simulink subsystem "PvtSubSys_LATC"  (R2020b)
settings: Solver=VariableStepAuto  StartTime=0.0  StopTime=10.0  RelTol=1e-3
values from neighbouring files (symbols this model uses):
  P_Global_CharSpd_ms : value not decoded    [PubParsGlobal.sldd]
  P_Global_SteeringAngleRatio : value not decoded    [PubParsGlobal.sldd]
  P_Global_WheelBase_m : value not decoded    [PubParsGlobal.sldd]
  P_LCS_A0_Limit = 0.25    [LATC.sldd]    (also in LCS_v05.sldd)
  P_LCS_A1_Limit = 0.002    [LATC.sldd]    (also in LCS_v05.sldd)
  P_LCS_communicationTest = 1.0    [LATC.sldd]    (also in LCS_v05.sldd)
  P_LCS_Current_Offset_Test_SW = 0.0    [LATC.sldd]
  P_LCS_Current_Offset_Test_Value = 0.0    [LATC.sldd]
  P_LCS_Curvature_bp : value not decoded    [LATC.sldd]
  P_LCS_CycleTime = 0.4 0.4 0.4 0.4 0.4 0.4 0.4 0.4 0.4 0.6 0.6 0.6 0.6 0.6 0.6 0.6 0.4 0.4 0.4 0.4 0.4 0.4 0.4 0.4 0.4 0.6 0.6 0.6 0.6 0.6 0.6 0.6 0.4 0.4 0.4 0.4 0.4 0.4 0.4 0.4 0.4 0.6 0.6 0.6 0.6 0.6 0.6 0.6 0.4 0.4 0.4 0.4 0.4 0.4 0.4 0.4 0.4 0.6 0.6 0.6 0.6 0.6 0.6 0.6 0.4 0.4 0.4 0.4 0.4 0.4 0.4 0.4 0.4 0.6 0.6 0.6 0.6 0.6 0.6 0.6 0.4 0.4 0.4 0.4 0.4 0.4 0.4 0.4 0.4 0.6 0.6 0.6 0.6 0.6 0.6 0.6 0.4 0.4 0.4 0.4    [LATC.sldd]
  P_LCS_ESS_AngleSlope_Limit = 2.9    [LATC.sldd]    (also in LCS_v05.sldd)
  P_LCS_IN_Offset_Test_SW = 0.0    [LATC.sldd]    (also in LCS_v05.sldd)
  P_LCS_IN_Offset_Test_Value = 0.0    [LATC.sldd]    (also in LCS_v05.sldd)
  P_LCS_LATC_CurOffsetVehicleSpdLimitValue_degs = 7.0    [LATC.sldd]
  P_LCS_LATC_Du_Max = 20.0    [LATC.sldd]
  P_LCS_LATC_ELKAngleSlope_ratio : value not decoded    [LATC.sldd]
  P_LCS_LATC_ELKMaxLatAcc_ms2 : value not decoded    [LATC.sldd]
  P_LCS_LATC_ESSAngleSlope_ratio : value not decoded    [LATC.sldd]
  P_LCS_LATC_ESSMaxLatAcc_ms2 : value not decoded    [LATC.sldd]
  P_LCS_LATC_LCAngleSlope_ratio : value not decoded    [LATC.sldd]
  P_LCS_LATC_LCCancleMaxLatAcc_ms2 : value not decoded    [LATC.sldd]
  P_LCS_LATC_LCEcoAngleSlope_ratio : value not decoded    [LATC.sldd]
  P_LCS_LATC_LCEcoMaxLatAcc_ms2 : value not decoded    [LATC.sldd]
  P_LCS_LATC_LCKAngleSlope_ratio : value not decoded    [LATC.sldd]
  P_LCS_LATC_LCKIEAngleSlope_ratio : value not decoded    [LATC.sldd]
  P_LCS_LATC_LCKIEMaxLatAcc_ms2 : value not decoded    [LATC.sldd]
  P_LCS_LATC_LCKMaxLatAcc_ms2 : value not decoded    [LATC.sldd]
  P_LCS_LATC_LCNormalAngleSlope_ratio : value not decoded    [LATC.sldd]
  P_LCS_LATC_LCNormalMaxLatAcc_ms2 : value not decoded    [LATC.sldd]
  P_LCS_LATC_LCSportAngleSlope_ratio : value not decoded    [LATC.sldd]
  P_LCS_LATC_LCSportMaxLatAcc_ms2 : value not decoded    [LATC.sldd]
  P_LCS_LATC_LKAAngleSlope_ratio : value not decoded    [LATC.sldd]
  P_LCS_LATC_LKAMaxLatAcc_ms2 : value not decoded    [LATC.sldd]
  P_LCS_LATC_MatrixQ1_st = 0.8 0.8 1.2 1.4 1.4 1.4 2.0 2.2 2.2 2.2 2.2 2.2 2.2 2.2 2.2 2.2 0.8 0.8 1.2 1.4 1.4 1.4 2.0 2.2 2.2 2.2 2.2 2.2 2.2 2.2 2.2 2.2 0.8 0.8 1.2 1.4 1.4 1.4 2.0 2.2 2.2 2.2 2.2 2.2 2.2 2.2 2.2 2.2 0.8 0.8 1.2 1.4 1.4 1.4 2.0 2.2 2.2 2.2 2.2 2.2 2.2 2.2 2.2 2.2 0.8 0.8 1.2 1.4 1.4 1.4 2.0 2.2 2.2 2.2 2.2 2.2 2.2 2.2 2.2 2.2 0.8 0.8 1.2 1.4 1.4 1.4 2.0 2.2 2.2 2.2 2.2 2.2 2.2 2.2 2.2 2.2 0.8 0.8 1.2 1.4    [LATC.sldd]
  P_LCS_LATC_MatrixQ3_st = 20.0 20.0 20.0 20.0 20.0 15.0 15.0 15.0 15.0 15.0 15.0 15.0 15.0 13.0 13.0 13.0 20.0 20.0 20.0 20.0 20.0 15.0 15.0 15.0 15.0 15.0 15.0 15.0 15.0 13.0 13.0 13.0 20.0 20.0 20.0 20.0 20.0 15.0 15.0 15.0 15.0 15.0 15.0 15.0 15.0 13.0 13.0 13.0 20.0 20.0 20.0 20.0 20.0 15.0 15.0 15.0 15.0 15.0 15.0 15.0 15.0 13.0 13.0 13.0 20.0 20.0 20.0 20.0 20.0 15.0 15.0 15.0 15.0 15.0 15.0 15.0 15.0 13.0 13.0 13.0    [LATC.sldd]
  P_LCS_LATC_MatrixR_st = 10.0 10.0 10.0 10.0 10.0 10.0 10.0 15.0 15.0 15.0 15.0 15.0 15.0 15.0 15.0 15.0 10.0 10.0 10.0 10.0 10.0 10.0 10.0 15.0 15.0 15.0 15.0 15.0 15.0 15.0 15.0 15.0 10.0 10.0 10.0 10.0 10.0 10.0 10.0 15.0 15.0 15.0 15.0 15.0 15.0 15.0 15.0 15.0 10.0 10.0 10.0 10.0 10.0 10.0 10.0 15.0 15.0 15.0 15.0 15.0 15.0 15.0 15.0 15.0 10.0 10.0 10.0 10.0 10.0 10.0 10.0 15.0 15.0 15.0 15.0 15.0 15.0 15.0 15.0 15.0    [LATC.sldd]
  P_LCS_LATC_Max_LatAcc = 4.0    [LATC.sldd]
  P_LCS_LATC_Max_Phi = 15.0    [LATC.sldd]
  P_LCS_LATC_Max_y = 0.5    [LATC.sldd]
  P_LCS_LATC_MPC_SW = 0.0    [LATC.sldd]
  P_LCS_LATC_PreView_SW = 1.0    [LATC.sldd]
  P_LCS_LATC_SoftConstWeight = 1.0    [LATC.sldd]
  P_LCS_LATC_StateActivAngleSlopeLimit_ratio : value not decoded    [LATC.sldd]
  P_LCS_LATC_StateActiveFlg_TabX_st : value not decoded    [LATC.sldd]
  P_LCS_LATC_StateActiveHoldTime_TabY_st : value not decoded    [LATC.sldd]
  P_LCS_LATC_StateHoldTime_st = 250.0    [LATC.sldd]
  P_LCS_LATC_TarAngleFliterWindowSize = 5.0    [LATC.sldd]
  P_LCS_LATC_TarAngleLP_Time = 0.02    [LATC.sldd]
  P_LCS_LATC_U_Max = 90.0    [LATC.sldd]
  P_LCS_LCK_AngleSlope_Limit = 1.4    [LATC.sldd]
  P_LCS_LineVaildSW = 0.0    [LATC.sldd]
  P_LCS_Lookahead_Distance : value not decoded    [LATC.sldd]
  P_LCS_Lookahead_DistanceFac : value not decoded    [LATC.sldd]
  P_LCS_PLAN_CurvePreView_s = 0.3    [LATC.sldd]
  P_LCS_PLAN_CurvePreview_TabX_m : value not decoded    [LATC.sldd]
  P_LCS_PLAN_CurvePreViewFilterTime_s = 0.1    [LATC.sldd]
  P_LCS_PLAN_ELKAyDtLimit_Tab_ms3 = 1.0 1.0 1.0 1.0 1.0 1.0 1.0 1.0 1.0 1.0 1.0 1.0 1.0 1.0 1.0 1.0 1.0 1.0 1.0 1.0 1.0 1.0 1.0 1.0 1.0 1.0 1.0 1.0 1.0 1.0 1.0 1.0 1.0 1.0 1.0 1.0 1.0 1.0 1.0 1.0 1.0 1.0 1.0 1.0 1.0 1.0 1.0 1.0 1.0 1.0 1.0 1.0 1.0 1.0 1.0 1.0 1.0 1.0 1.0 1.0 1.0 1.0 1.0 1.0 1.0 1.0 1.0 1.0 1.0 1.0 1.0 1.0 1.0 1.0 1.0 1.0 1.0 1.0 1.0 1.0 1.0 1.0 1.0 1.0 1.0 1.0 1.0 1.0 1.0 1.0 1.0 1.0 1.0 1.0 1.0 1.0 1.0 1.0 1.0 1.0    [LATC.sldd]
  P_LCS_PLAN_ESSAyDtLimit_Tab_ms3 = 1.0 1.0 1.0 1.0 1.0 1.0 1.0 1.0 1.0 1.0 1.0 1.0 1.0 1.0 1.0 1.0 1.0 1.0 1.0 1.0 1.0 1.0 1.0 1.0 1.0 1.0 1.0 1.0 1.0 1.0 1.0 1.0 1.0 1.0 1.0 1.0 1.0 1.0 1.0 1.0 1.0 1.0 1.0 1.0 1.0 1.0 1.0 1.0 1.0 1.0 1.0 1.0 1.0 1.0 1.0 1.0 1.0 1.0 1.0 1.0 1.0 1.0 1.0 1.0 1.0 1.0 1.0 1.0 1.0 1.0 1.0 1.0 1.0 1.0 1.0 1.0 1.0 1.0 1.0 1.0 1.0 1.0 1.0 1.0 1.0 1.0 1.0 1.0 1.0 1.0 1.0 1.0 1.0 1.0 1.0 1.0 1.0 1.0 1.0 1.0    [LATC.sldd]
  P_LCS_PLAN_LCCancleAyDtLimit_Tab_ms3 = 1.0 1.0 1.0 1.0 1.0 1.0 1.0 1.0 1.0 1.0 1.0 1.0 1.0 1.0 1.0 1.0 1.0 1.0 1.0 1.0 1.0 1.0 1.0 1.0 1.0 1.0 1.0 1.0 1.0 1.0 1.0 1.0 1.0 1.0 1.0 1.0 1.0 1.0 1.0 1.0 1.0 1.0 1.0 1.0 1.0 1.0 1.0 1.0 1.0 1.0 1.0 1.0 1.0 1.0 1.0 1.0 1.0 1.0 1.0 1.0 1.0 1.0 1.0 1.0 1.0 1.0 1.0 1.0 1.0 1.0 1.0 1.0 1.0 1.0 1.0 1.0 1.0 1.0 1.0 1.0 1.0 1.0 1.0 1.0 1.0 1.0 1.0 1.0 1.0 1.0 1.0 1.0 1.0 1.0 1.0 1.0 1.0 1.0 1.0 1.0    [LATC.sldd]
  P_LCS_PLAN_LCEcoAyDtLimit_Tab_ms3 = 1.0 1.0 1.0 1.0 1.0 1.0 1.0 1.0 1.0 1.0 1.0 1.0 1.0 1.0 1.0 1.0 1.0 1.0 1.0 1.0 1.0 1.0 1.0 1.0 1.0 1.0 1.0 1.0 1.0 1.0 1.0 1.0 1.0 1.0 1.0 1.0 1.0 1.0 1.0 1.0 1.0 1.0 1.0 1.0 1.0 1.0 1.0 1.0 1.0 1.0 1.0 1.0 1.0 1.0 1.0 1.0 1.0 1.0 1.0 1.0 1.0 1.0 1.0 1.0 1.0 1.0 1.0 1.0 1.0 1.0 1.0 1.0 1.0 1.0 1.0 1.0 1.0 1.0 1.0 1.0 1.0 1.0 1.0 1.0 1.0 1.0 1.0 1.0 1.0 1.0 1.0 1.0 1.0 1.0 1.0 1.0 1.0 1.0 1.0 1.0    [LATC.sldd]
  P_LCS_PLAN_LCKAyDtLimit_Tab_ms3 = 1.5 1.5 1.5 1.5 1.5 1.5 1.5 1.5 1.5 1.5 1.5 1.5 1.5 1.5 1.5 1.5 1.5 1.5 1.5 1.5 1.5 1.5 1.5 1.5 1.5 1.5 1.5 1.5 1.5 1.5 1.5 1.5 1.5 1.5 1.5 1.5 1.5 1.5 1.5 1.5 1.5 1.5 1.5 1.5 1.5 1.5 1.5 1.5 1.5 1.5 1.5 1.5 1.5 1.5 1.5 1.5 1.5 1.5 1.5 1.5 1.5 1.5 1.5 1.5 1.5 1.5 1.5 1.5 1.5 1.5 1.5 1.5 1.5 1.5 1.5 1.5 1.5 1.5 1.5 1.5 1.5 1.5 1.5 1.5 1.5 1.5 1.5 1.5 1.5 1.5 1.5 1.5 1.5 1.5 1.5 1.5 1.5 1.5 1.5 1.5    [LATC.sldd]
  P_LCS_PLAN_LCKIEAyDtLimit_Tab_ms3 = 1.0 1.0 1.0 1.0 1.0 1.0 1.0 1.0 1.0 1.0 1.0 1.0 1.0 1.0 1.0 1.0 1.0 1.0 1.0 1.0 1.0 1.0 1.0 1.0 1.0 1.0 1.0 1.0 1.0 1.0 1.0 1.0 1.0 1.0 1.0 1.0 1.0 1.0 1.0 1.0 1.0 1.0 1.0 1.0 1.0 1.0 1.0 1.0 1.0 1.0 1.0 1.0 1.0 1.0 1.0 1.0 1.0 1.0 1.0 1.0 1.0 1.0 1.0 1.0 1.0 1.0 1.0 1.0 1.0 1.0 1.0 1.0 1.0 1.0 1.0 1.0 1.0 1.0 1.0 1.0 1.0 1.0 1.0 1.0 1.0 1.0 1.0 1.0 1.0 1.0 1.0 1.0 1.0 1.0 1.0 1.0 1.0 1.0 1.0 1.0    [LATC.sldd]
  P_LCS_PLAN_LCNormalAyDtLimit_Tab_ms3 = 1.0 1.0 1.0 1.0 1.0 1.0 1.0 1.0 1.0 1.0 1.0 1.0 1.0 1.0 1.0 1.0 1.0 1.0 1.0 1.0 1.0 1.0 1.0 1.0 1.0 1.0 1.0 1.0 1.0 1.0 1.0 1.0 1.0 1.0 1.0 1.0 1.0 1.0 1.0 1.0 1.0 1.0 1.0 1.0 1.0 1.0 1.0 1.0 1.0 1.0 1.0 1.0 1.0 1.0 1.0 1.0 1.0 1.0 1.0 1.0 1.0 1.0 1.0 1.0 1.0 1.0 1.0 1.0 1.0 1.0 1.0 1.0 1.0 1.0 1.0 1.0 1.0 1.0 1.0 1.0 1.0 1.0 1.0 1.0 1.0 1.0 1.0 1.0 1.0 1.0 1.0 1.0 1.0 1.0 1.0 1.0 1.0 1.0 1.0 1.0    [LATC.sldd]
  P_LCS_PLAN_LCSportAyDtLimit_Tab_ms3 = 1.0 1.0 1.0 1.0 1.0 1.0 1.0 1.0 1.0 1.0 1.0 1.0 1.0 1.0 1.0 1.0 1.0 1.0 1.0 1.0 1.0 1.0 1.0 1.0 1.0 1.0 1.0 1.0 1.0 1.0 1.0 1.0 1.0 1.0 1.0 1.0 1.0 1.0 1.0 1.0 1.0 1.0 1.0 1.0 1.0 1.0 1.0 1.0 1.0 1.0 1.0 1.0 1.0 1.0 1.0 1.0 1.0 1.0 1.0 1.0 1.0 1.0 1.0 1.0 1.0 1.0 1.0 1.0 1.0 1.0 1.0 1.0 1.0 1.0 1.0 1.0 1.0 1.0 1.0 1.0 1.0 1.0 1.0 1.0 1.0 1.0 1.0 1.0 1.0 1.0 1.0 1.0 1.0 1.0 1.0 1.0 1.0 1.0 1.0 1.0    [LATC.sldd]
  P_LCS_PLAN_LKAAyDtLimit_Tab_ms3 = 1.0 1.0 1.0 1.0 1.0 1.0 1.0 1.0 1.0 1.0 1.0 1.0 1.0 1.0 1.0 1.0 1.0 1.0 1.0 1.0 1.0 1.0 1.0 1.0 1.0 1.0 1.0 1.0 1.0 1.0 1.0 1.0 1.0 1.0 1.0 1.0 1.0 1.0 1.0 1.0 1.0 1.0 1.0 1.0 1.0 1.0 1.0 1.0 1.0 1.0 1.0 1.0 1.0 1.0 1.0 1.0 1.0 1.0 1.0 1.0 1.0 1.0 1.0 1.0 1.0 1.0 1.0 1.0 1.0 1.0 1.0 1.0 1.0 1.0 1.0 1.0 1.0 1.0 1.0 1.0 1.0 1.0 1.0 1.0 1.0 1.0 1.0 1.0 1.0 1.0 1.0 1.0 1.0 1.0 1.0 1.0 1.0 1.0 1.0 1.0    [LATC.sldd]
  P_LCS_PLAN_MinPlanDis_m : value not decoded    [LATC.sldd]
  P_LCS_PLAN_PreCurMinDisFac_ratio : value not decoded    [LATC.sldd]
  P_LCS_PLAN_PreDisCurve_TabX_m : value not decoded    [LATC.sldd]
  P_LCS_PLAN_StateActiv_AyDtLimit_ms3 : value not decoded    [LATC.sldd]
  P_LCS_PLAN_VehicleSpd_TabX_kph : value not decoded    [LATC.sldd]
  P_LCS_PLAN_VehicleSpd_TabY_Kph : value not decoded    [LATC.sldd]
  P_LCS_Trq_Switch = 0.0    [LATC.sldd]    (also in LCS_v05.sldd)
  P_LCS_VehicleSpd_TabX_Kph : value not decoded    [LATC.sldd]
undefined symbols (not defined in the file or in its folder): HWP_AngCmdReqVal, HWP_AngCmdReqValVld, HWP_FuncTrqCmdReqFlag, HWP_ReqCtrlEPS, HWP_ReqCtrlEPSVld, HWP_TrqOvlCmdReqValue, HWP_WorkReq, HWP_WorkReqVld
libraries: simulink x4, dspbuff3 x2
(part 6 of 8)

== matlab function PvtSubSys_LATC/LATC/LateralControl/LCS_Angle/Controller/TargetAngleCalc/TarSteerAngleCalc ==
  data: Final_steer_angle_cmd output; LatError_contribution output; LatErrorRate_contribution output; HeadingError_contribution output; HeadingErrorRate_contribution output; ControlValid input; SteerAngle input; CurrentSteerAngleOffset input; steer_angle_cmd output size=[1,1]; vy input; vx input; phi input; phi_dot input; TarTraj_x input size=[100 1]; TarTraj_y input size=[100 1]; Left_steer_ratio input; Right_steer_ratio input; Matrix_q1 input; Matrix_q2 input; Matrix_R input; Max_Phi input; Max_y input; U_Max input; Du_Max input; Max_LatAcc input; SoftConstWeight input
function [Final_steer_angle_cmd,LatError_contribution,LatErrorRate_contribution,...
    HeadingError_contribution,HeadingErrorRate_contribution,steer_angle_cmd]= ...
    MPC_ReferenceTrajectory_Algorithm(ControlValid,SteerAngle,CurrentSteerAngleOffset,vy,vx,phi,phi_dot,TarTraj_x,TarTraj_y,...
    Left_steer_ratio,Right_steer_ratio,Matrix_q1,Matrix_q2,Matrix_R,Max_Phi,Max_y,U_Max,Du_Max,Max_LatAcc,SoftConstWeight)

LatError_contribution = single(0);
LatErrorRate_contribution = single(0);
HeadingError_contribution = single(0);
HeadingErrorRate_contribution = single(0);
if ControlValid
    %% 1.车辆参数
    %1.1 车的大小及长度参数
    veh_params.vehicle_length = single(4.875);
    veh_params.vehicle_width  = single(2.2);
    veh_params.vehicle_height = single(1.69);
    %1.2 车辆控制参数
    veh_params.wheel_base = single(2.92);               %轴距, m
    veh_params.Vch = single(23.5);                      %特征车速
    veh_params.mu = single(0.85);                       %路面摩擦限制
    veh_params.max_acceleration = single(2);            %车辆最大加速度
    veh_params.max_deceleration = single(-2);           %车辆最大减速度
    veh_params.left_steer_ratio = Left_steer_ratio;     %车辆左侧转向传动比%
    veh_params.right_steer_ratio = Right_steer_ratio;   %车辆右侧转向传动比%
    veh_params.cf = single(55000);                      %车辆前轮侧偏刚度N/rad(两侧轮胎等效为一个*2)
    veh_params.cr = single(55000);                      %车辆后轮侧偏刚度N/rad
    veh_params.clf = single(5000);                      %车辆前轮纵向刚度(两侧轮胎等效为一个*2)
    veh_params.clr = single(5000);                      %车辆后轮纵向刚度
    
    veh_params.mass_fl = single(520);                   %车辆左前轮负重
    veh_params.mass_fr = single(520);                   %车辆右前轮负重
    veh_params.mass_rl = single(520);                   %车辆左后轮负重
    veh_params.mass_rr = single(520);                   %车辆右后轮负重
    veh_params.Sf = single(0.2);                        %车辆前轮滑移率
    veh_params.Sr = single(0.2);                        %车辆后轮滑移率
    %1.3 方向盘转角转换为车轮转角+度转弧度
    if (SteerAngle>=single(0))
        steer_transmission_ratio = veh_params.left_steer_ratio;
    else
        steer_transmission_ratio = veh_params.right_steer_ratio;
    end
    % FrontWheel_AngleK1_rad = steer_angleK1 / (single(57.3) * steer_transmission_ratio);%反算前轮转角并转换成弧度制 上一帧请求值
    FrontWheel_AngleK1_rad = SteerAngle/(single(57.3) * steer_transmission_ratio); %反算前轮转角并转换成弧度制
   %% 2.控制参数计算
    mass_front =  veh_params.mass_fl + veh_params.mass_fr;
    mass_rear  =  veh_params.mass_rl + veh_params.mass_rr;
    mass =  mass_front + mass_rear;
    lf = veh_params.wheel_base * (single(1.0) - mass_front / mass);% distance from front tires to cg, m 前轴到质心的距离
    lr = veh_params.wheel_base * (single(1.0) - mass_rear / mass);% distance from rear tires to cg, m  后轴到质心的距离
    iz = lf * lf * mass_front + lr * lr * mass_rear; % 转动惯量
    %---------------------------求车辆响应增益---------------------------%
    % % 车辆模型，状态为[beta,wr]
    % 求车辆响应增益
    Veh_Speed = (max(vx, single(0.2)));
    AAr = [(veh_params.cf+veh_params.cr),((veh_params.cf*lf-veh_params.cr*lr)/Veh_Speed)+mass*Veh_Speed;
           (veh_params.cf*lf-veh_params.cr*lr),(veh_params.cf*lf^2+veh_params.cr*lr^2)/Veh_Speed];
    BBr = [veh_params.cf;veh_params.cf*lf];
    a11 = AAr(1,1);
    a12 = AAr(1,2);
    a21 = AAr(2,1);
    a22 = AAr(2,2);
    b1 = BBr(1);
    b2 = BBr(2);
    %Ta = a11+a22;
    Da = a11*a22-a12*a21;
    
    Gr = (b2.*a11-b1.*a21)./Da;   % 稳态横摆角速度增益，理想化增益是偏大，因为轮胎侧偏刚度会变小
    % Gb = (b1.*a22-b2.*a12)./Da; % 稳态质心侧偏角增益，理想化增益是偏大，因为轮胎侧偏刚度会变小
    Gay = Gr*Veh_Speed;           % 稳态侧向加速度增益，理想化增益是偏大，因为轮胎侧偏刚度会变小
   %% 3.mpc算法
   % ----------------------车辆动力学模型--------------------------------%
   % 状态量=[y_dot,x_dot,phi,phi_dot,Y,X]，控制量为前轮偏角delta_f
   % dy_dot=-x_dot*phi_dot+2*(Ccf*(delta_f-(y_dot+a*phi_dot)/x_dot)+Ccr*(b*phi_dot-y_dot)/x_dot)/m;
   % dx_dot=y_dot*phi_dot+2*(Clf*Sf+Clr*Sr-Ccf*delta_f*(delta_f-(y_dot+phi_dot*a)/x_dot))/m;
   % dphi_dot=dphi_dot;
   % dphi_dot=(2*a*Ccf*(delta_f-(y_dot+a*phi_dot)/x_dot)-2*b*Ccr*(b*phi_dot-y_dot)/x_dot)/I;
   % Y_dot=x_dot*sin(phi)+y_dot*cos(phi);
   % X_dot=x_dot*cos(phi)-y_dot*sin(phi);
   % 通过Matlab求雅克比矩阵
   % 雅克比矩阵求解
   % f=[dy_dot;dx_dot;phi_dot;dphi_dot;Y_dot;X_dot];%动力学模型
   % kesi=[y_dot,x_dot,phi,phi_dot,Y,X];%系统状态量
   % v=delta_f;
   % R=jacobian(f,kesi);%矩阵A(t)-连续
   % R2=jacobian(f,v);%矩阵B(t)-连续
    A =  [-((2*veh_params.cf)/vx+(2*veh_params.cr)/vx)/mass   ((2*veh_params.cf*(vy+lf*phi_dot))/vx^2+(2*veh_params.cr*(vy-lr*phi_dot))/vx^2)/mass-phi_dot   0   -vx-((2*veh_params.cf*lf)/vx-(2*veh_params.cr*lr)/vx)/mass   0   0;
          phi_dot + (2*veh_params.cf*FrontWheel_AngleK1_rad)/(mass*vx)       -(2*veh_params.cf*FrontWheel_AngleK1_rad*(vy + lf*phi_dot))/(mass*vx^2)         0   vy + (2*veh_params.cf*lf*FrontWheel_AngleK1_rad)/(mass*vx)   0   0;
          0                                                    0                                                                                             0   1                                                            0   0;
    -((2*veh_params.cf*lf)/vx-(2*veh_params.cr*lr)/vx)/iz   ((2*veh_params.cf*lf*(vy+lf*phi_dot))/vx^2-(2*veh_params.cr*lr*(vy-lr*phi_dot))/vx^2)/iz         0   -((2*veh_params.cf*lf^2)/vx + (2*veh_params.cr*lr^2)/vx)/iz  0   0;
          cos(phi)                                              sin(phi)                                                                     vx*cos(phi)-vy*sin(phi)              0                                           0   0;
          -sin(phi)                                             cos(phi)                                                                     -vy*cos(phi)-vx*sin(phi)             0                                           0   0;
          ];
    B = [(2*veh_params.cf)/mass;
         -(2*veh_params.cf*FrontWheel_AngleK1_rad+2*veh_params.cf*(FrontWheel_AngleK1_rad-(vy+lf*phi_dot)/vx))/mass;
         0;
         (2*veh_params.cf*lf)/iz;
         0;
         0;];
     %-------------------状态方程离散化----------------------------------%
     % 控制矩阵求解(将连续矩阵转换为离散矩阵，采用近似算法  A=I+T*A(t),B=T*B(t))
     Ts = single(0.02);
     [A_row,~] = size(A);% 6*6
     Ad = single((eye(A_row)+A*Ts/2)/(eye(A_row)-A*Ts/2)); %6*6
     %Ad = single((eye(A_row)+A*Ts)); %6*6
     Bd = single(Ts*B);% 6*1
     %-------------------------------------%
     Nx=6;%状态量的个数
     Nu=1;%控制量的个数
     Ny=2;%输出量的个数
     Np = 10;%预测步长
     Nc= 3;%控制步长
    %-----------------------------------------------------------------%
    % 状态量=[y_dot,x_dot,phi,phi_dot,Y,X]
    Q = single(zeros(Ny,Ny));                %  phi Y
    Q(1,1) = Matrix_q1;                      %调整q矩阵的 Q为状态权重系数
    Q(2,2) = Matrix_q2;
    % R = single(zeros(1,1));
    R = Matrix_R;                            %R为控制量权重系数 R=1
    %-------------------状态矩阵构建----------------------------------%
    %  以下计算kesi,即状态量与控制量合在一起,变成增量形式
    kesi=zeros(Nx+Nu,1);
    kesi(1)=vy;  % CarSim输出的是km/h，转换为m/s
    kesi(2)=vx;  % CarSim输出的是km/h，转换为m/s
    kesi(3)=phi; % CarSim输出的为角度，角度转换为弧度
    kesi(4)=phi_dot; % CarSim输出的为角度，角度转换为弧度
    kesi(5)=0; %单位为m 因为全局坐标系固结与车辆坐标系上因此X Y = 0
    kesi(6)=0;
    kesi(7)=FrontWheel_AngleK1_rad;
    Y=0;%起始点在全局坐标系的位置
    X=0;%起始点在全局坐标系的位置
    %-----------------------权重矩阵生成-----------------------------%
    % 注意这个Q，如果没有输出矩阵C，这个位置Q有可能也需要增广
    Qt = single(zeros(Np*Ny,Np*Ny));
    for r = 1:Np
        for c = 1:Np
            if r ==c
                Qt(((r-1)*Ny)+1:r*Ny,((r-1)*Ny)+1:r*Ny) = Q; % 20*20
            end
        end
    end
    Rt = single(zeros(Nc*Nu,Nc*Nu));%
    for i = 1:Nc
        for j = 1:Nc
            if i==j
                Rt(((i-1)*Nu)+1:i*Nu,((i-1)*Nu)+1:i*Nu) = R; % 10*10
            end
        end
    end
    %--------以下为根据非线性模型预测下一时刻状态量，通过离散模型与非线性模型做差计算出高阶项的误差，作为模型的扰动项---------%
    % d_k=zeros(Nx,1); % 计算偏差 6*1
    state_k1=zeros(Nx,1);% 预测的下一时刻状态量，用于计算偏差 6*1
    state_k1(1,1)=vy+Ts*(-vx*phi_dot+2*(veh_params.cf*(FrontWheel_AngleK1_rad-(vy+lf*phi_dot)/vx)+veh_params.cr*(lr*phi_dot-vy)/vx)/mass);
    state_k1(2,1)=vx+Ts*(vy*phi_dot+2*(veh_params.clf*veh_params.Sf+veh_params.clr*veh_params.Sr-veh_params.cf*FrontWheel_AngleK1_rad*(FrontWheel_AngleK1_rad-(vy+phi_dot*lf)/vx))/mass);
    state_k1(3,1)=phi+Ts*phi_dot;
    state_k1(4,1)=phi_dot+Ts*((2*lf*veh_params.cf*(FrontWheel_AngleK1_rad-(vy+lf*phi_dot)/vx)-2*lr*veh_params.cr*(lr*phi_dot-vy)/vx)/iz);
    state_k1(5,1)=Y+Ts*(vx*sin(phi)+vy*cos(phi));
    state_k1(6,1)=X+Ts*(vx*cos(phi)-vy*sin(phi));
    %-------------求偏差，作为扰动或者未知项------------------------------%
    d_k=state_k1-Ad*kesi(1:6,1)-Bd*kesi(7,1);%根据falcone公式（2.11b）求得d(k,t) 6*1-6*1-6*1
    %--------------对偏差扰动项做增广-------------------------------------%
    d_piao_k=zeros(Nx+Nu,1);%d_k的增广形式，参考falcone(B,4c) 7*1
    d_piao_k(1:6,1)=d_k;
    d_piao_k(7,1)=0;
    %----------------扩展状态矩阵，将输入由绝对量变为增量----------------%
    Ae = [Ad,Bd;zeros(Nu,Nx),eye(Nu)]; % 7*7
    Be = [Bd;eye(Nu)]; % 7*1
    %----------------输出预测矩阵构建-----------------------------------%
    C=[0 0 1 0 0 0 0;  % kesi=[y_dot,x_dot,phi,phi_dot,Y,X];%系统状态量
       0 0 0 0 1 0 0;];% 这是和输出量紧密关联的 2*7,输出 phi Y X
    [CAe_row,CAe_col] = size(C*Ae); % 2*7
    [CBe_row,CBe_col] = size(C*Be); % 2*1
    [C_row,C_col] = size(C); % 2*7
    [d_piao_row,d_piao_col] = size(d_piao_k); % 7*1
    
    At = single(zeros(Np*CAe_row,CAe_col)); % 20*7
    Bt_c = single(zeros(Np*C_row,Np*CBe_col)); % 20*10
    Bt_c_temp = single(zeros(C_row,Np*CBe_col)); % 2*10
    Dt = single(zeros(Np*d_piao_row,d_piao_col)); % 70*1
    Et = single(zeros(Np*C_row,Np*C_col)); % 20*70
    Et_temp = single(zeros(C_row,Np*C_col));% 2*70
    for r=1:Np
        Dt(((r-1)*d_piao_row+1):r*d_piao_row,:) = d_piao_k;%理论上来说，这个是要实时更新的，但是为了简便这里近似
        At(((r-1)*CAe_row+1):r*CAe_row,:) = C*Ae^r;
        for c=1:Np
            if c<=r
                Bt_c_temp(:,((c-1)*CBe_col+1):c*CBe_col) = C*Ae^(r-c)*Be;%2*1
                Et_temp(:,((c-1)*C_col+1):c*C_col) = C*Ae^(r-c);
            end
        end
        Bt_c(((r-1)*CBe_row+1):r*CBe_row,:) = Bt_c_temp;
        Et(((r-1)*CAe_row+1):r*CAe_row,:) = Et_temp;
    end
    Bt = Bt_c(:,1:Nu*Nc);
    %-----------------转换后的优化目标函数矩阵-----------------------%
    Row = SoftConstWeight;%松弛因子权重
    H=[Bt'*Qt*Bt+Rt,zeros(Nu*Nc,1);zeros(1,Nu*Nc),Row]; % Row 
    %-----------------算f矩阵中与参考的误差-------------------------%
    %计算预测输出
    X_predict=zeros(Np,1);%用于保存预测时域内的纵向位置信息，这是计算期望轨迹的基础
    
    phi_ref=zeros(Np,1);%用于保存预测时域内的期望轨迹
    Y_ref=zeros(Np,1);%用于保存预测时域内的期望轨迹
    % C = fitting(TarTraj_x,TarTraj_y);
    XX = [TarTraj_x(1,1) TarTraj_x(10,1) TarTraj_x(30,1) TarTraj_x(60,1)];
    YY = [TarTraj_y(1,1) TarTraj_y(10,1) TarTraj_y(30,1) TarTraj_y(60,1)];
    [A,B,CC,D] = pl(XX,YY);
    % C0 = C(1);C1 = C(2);C2 = C(3);C3 = C(4);
    C0 = D;C1 = CC;C2 = B;C3 = A;
    for i=1:1:Np
        X_DOT=vx*cos(phi)-vy*sin(phi);%惯性坐标系下纵向速度
        X_predict(i,1)=X+X_DOT*i*Ts;%首先计算出未来X的位置，X(t)=X+X_dot*t

        Y_ref(i,1) =  C3* X_predict(i,1)^3 +  C2*X_predict(i,1)^2 +  C1*X_predict(i,1) +  C0;
        phi_ref(i,1) = atan( C3* X_predict(i,1)^2 +  C2*X_predict(i,1) +  C1); 
    end
    State_ref=[phi_ref;Y_ref];
    %---------------------------------------------------------------%
    State_Error = State_ref-At*kesi-Et*Dt;
    F=[-1*Bt'*Qt*State_Error;0];
    %--------------------------约束矩阵生成--------------------------------%
    %控制量约束
    A_t=zeros(Nc,Nc);%见falcone论文 P181
    for p=1:1:Nc
        for q=1:1:Nc
            if q<=p 
                A_t(p,q)=1;
            else 
                A_t(p,q)=0;
            end
        end 
    end 
    A_I=kron(A_t,eye(Nu));%求克罗内克积
    Ut=kron(ones(Nc,1),FrontWheel_AngleK1_rad);
    
    U_Max_rad = U_Max/single(57.3); % U_Max deg
    Du_Max_rad = Du_Max*Ts/single(57.3); % Du_Max deg/s
    
    umin = -U_Max_rad;% 最大方向盘转角rad
    umax = U_Max_rad;
    delta_umin = -Du_Max_rad;
    delta_umax = Du_Max_rad;
    Umin=kron(ones(Nc,1),umin);
    Umax=kron(ones(Nc,1),umax);
    
    %输出量约束
    % ycmax=[0.21;5];
    % ycmin=[-0.3;-3];
    Max_Phi_rad = Max_Phi/single(57.3);
    ycmax=[Max_Phi_rad;Max_y]; % 最大朝向角与最大横向偏差，因为车体坐标与全局坐标重合，因此可以理解为最大的朝向角偏差和横向位置偏差 rad m
    ycmin=[-Max_Phi_rad;-Max_y];
    Ycmax=kron(ones(Np,1),ycmax);
    Ycmin=kron(ones(Np,1),ycmin);
    
    %结合控制量约束和输出量约束
    A_cons =[A_I zeros(Nu*Nc,1);-A_I zeros(Nu*Nc,1);Bt zeros(Ny*Np,1);-Bt zeros(Ny*Np,1)];%（求解方程）状态量不等式约束增益矩阵，转换为绝对值的取值范围
    b_cons =[Umax-Ut;-Umin+Ut;Ycmax-At*kesi-Et*Dt;-Ycmin+At*kesi+Et*Dt];%（求解方程）状态量不等式约束的取值
    % 增加软约束，希望侧向加速度<4m/s^2，否则增加惩罚
    Ay_softbound = Max_LatAcc;% 为了舒适性，希望侧向加速度<4m/s^2，否则增加惩罚
    Ay_SoftBound=kron(ones(Nc,1),Ay_softbound); 
    A_cons1 = [Gay*eye(Nu*Nc)*A_I,-ones(Nu*Nc,1);-Gay*eye(Nu*Nc)*A_I,-ones(Nu*Nc,1)];% Gay*Delta_UK1-epsilon; -Gay*Delta_UK1-epsilon
    Delta_UK1 = kron(ones(Nc,1), FrontWheel_AngleK1_rad);%上一帧的前轮转角
    b_cons1 = [Ay_SoftBound-Gay*eye(Nu*Nc)*Delta_UK1;Ay_SoftBound+Gay*eye(Nu*Nc)*Delta_UK1];
    % 不等式约束合成
    A_cons = [A_cons;A_cons1];
    b_cons = [b_cons;b_cons1];

    %状态量约束
    mu = single(0.85);
    g = single(9.8);
    delta_Umin=kron(ones(Nc,1),delta_umin);
    delta_Umax=kron(ones(Nc,1),delta_umax);
    lb=[delta_Umin;0];%（求解方程）状态量下界，包含控制时域内控制增量和松弛因子
    ub=[delta_Umax;mu*g-Ay_softbound];%（求解方程）状态量上界，包含控制时域内控制增量和松弛因子
    
    A_cons = [A_cons;eye((Nc*Nu)+1);-eye((Nc*Nu)+1)];
    b_cons = [b_cons;ub;-lb];
    
    %-------------------QP问题求解------------------------%
    % min(J) = 0.5x'Hx + f'x  
    % A_Const*x <= b
    uDelta = MPC_Solver_QPhild(H,F,A_cons,b_cons);% 增加了软约束的变量
    
    FrontWheel_Angle = FrontWheel_AngleK1_rad +uDelta(1); % 取第一个值作为输入
    %--------------前转角反算方向盘转角+弧度转角度---------------------%
    if (FrontWheel_Angle>=0)
        steer_transmission_ratio = veh_params.left_steer_ratio;
    else
        steer_transmission_ratio = veh_params.right_steer_ratio;
    end
    Final_steer_angle_cmd = FrontWheel_Angle * single(57.3) * steer_transmission_ratio; 
    % 反算方向盘转角并转换为角度制deg,输出算法计算角度作为观测，下一步会补偿转向不足。
    steer_angle_cmd = Final_steer_angle_cmd + single(CurrentSteerAngleOffset); % 后期会补充转向不足
    
else
    steer_angle_cmd = SteerAngle;
    Final_steer_angle_cmd = single(0);
    LatError_contribution = single(0);
    LatErrorRate_contribution = single(0);
    HeadingError_contribution = single(0);
    HeadingErrorRate_contribution = single(0);
end
end
function eta = MPC_Solver_QPhild(H,f,A_Const,b)
% 二次规划
% 该算法是原始对偶算法，该方法充分的剖析了优化问题的结构，是求解二次规划问题的一个较好的算法。
% J = 0.5x'Hx + f'x = min
% A_Const*x <= b
[n1,~] = size(A_Const);
eta = -H\f;
kk = single(0);
for i = 1:n1
    if(A_Const(i,:)*eta>b(i))
        kk = kk+single(1);
    else
        kk = kk+single(0);
    end
end
if kk == 0
    return;
end
P = A_Const*(H\A_Const');
d = (A_Const*(H\f)+b);
[n,m] = size(d);
x_ini = zeros(n,m);
lambda = x_ini;
for km = 1:38
    lambda_p = lambda;
    for i = 1:n
        w = P(i,:)*lambda - P(i,i)*lambda(i,1);
        w = w + d(i,1);
        la = -w/P(i,i);
        lambda(i,1) = max(0,la);
    end
    al = (lambda - lambda_p)'*(lambda - lambda_p);
    if(al<10e-8)
        break
    end
end
eta = -H\f -H\A_Const'*lambda;
end
function [E]=fitting(F1,F2)%最小二乘法拟合
A1=double(zeros(4));
B1=double(zeros(4,1));
m=length(F1)-1;
for j1=uint8(1):uint8(1):uint8(4)
    for i1=uint8(1):uint8(1):uint8(4)
        for k1=1:1:m+1
            A1(j1,i1)=A1(j1,i1)+F1(k1)^single(i1+j1-2);
        end
    end
end

for j1=uint8(1):uint8(1):uint8(4)
    for i1=1:1:m+1
        B1(j1)=B1(j1)+F2(i1)*F1(i1)^single(j1-1);
    end
end
E=A1\B1;
end
function [A,B,C,D] = pl(X,Y)
MatrixA = [X(1)^3,X(1)^2,X(1),1;...
           X(2)^3,X(2)^2,X(2),1;...
           X(3)^3,X(3)^2,X(3),1;...
           X(4)^3,X(4)^2,X(4),1];
MatrixB = [Y(1);Y(2);Y(3);Y(4)];
if det(MatrixA)==0
    A=cast(0,class(X(1)));
    B=cast(0,class(X(1)));
    C=cast(0,class(X(1)));
    D=cast(0,class(X(1)));
else
    P = MatrixA\MatrixB;
    A = P(1);
    B = P(2);
    C = P(3);
    D = P(4);
end
% coder.allowpcode('plain');
end

== matlab function PvtSubSys_LATC/communicationTest4/MATLAB Function1 ==
  data: uint8outK1 input uint8; uint8out output uint8; countk1 input uint8; count output uint8
function [uint8out,count] = uint8(uint8outK1,countk1)
count=countk1+uint8(1);
uint8out=uint8outK1;
if count>=100
    count=uint8(0);
end
if count==99
    uint8out=uint8outK1+uint8(1);
    if uint8out>2
        uint8out=uint8(0);
    end      
end

== matlab function PvtSubSys_LATC/communicationTest4/MATLAB Function2 ==
  data: factor input single; singlemin input single; singlemax input single; singleoutK1 input single; singleout output single; countk1 input uint8; count output uint8
function [singleout,count] = single(factor,singlemin,singlemax,singleoutK1,countk1)
count=countk1+uint8(1);
singleout=singleoutK1;
if count>=100
    count=uint8(0);
end
if count==99
    singleout=singleoutK1+factor;
    if singleout>singlemax
        singleout=singlemin;
    end      
end

== matlab function PvtSubSys_LATC/LATC/LateralControl/LCS_Angle/Controller/TargetAngleCalc/MATLAB Function3 ==
  data: Speed_ms input; Vy_SteerAngle_Vch output; SteerWheelAngle input; YawRate input; Vy_SteerAngle_Kv output; Vy_YawRate output; Critical_Spd output; CharSpd output; SteerChar output; Vch_Cal output
function [Vy_SteerAngle_Vch,Vy_SteerAngle_Kv,Vy_YawRate,Critical_Spd,CharSpd,SteerChar,Vch_Cal]= Vy_Calc(Speed_ms,SteerWheelAngle,YawRate)
    m = single(1720);
    L=single(2.91);
    a = single(1.27);
    b = single(1.64);
    Vch=single(23.5);
    caf = single(2*55000);
    car = single(2*75000);
    %%  根据Vy/steerAngle = K_gain，其中Kv(不足转向斜率)根据特征车速计算
    KKg1 = (Vch*Vch*Speed_ms)/((Vch^2+Vch^2)*L);
    KKg2 = (b - ((m*a*Speed_ms*Speed_ms)/(car*L)));
    K_gain = KKg1*KKg2;
    Vy_SteerAngle_Vch = (SteerWheelAngle/15.5/57.3)*K_gain;
    %%  根据Vy/steerAngle = KK_gain，其中Kv(不足转向斜率)根据前后轮胎刚度计算
    Kg1 = (car*caf*b*L*Speed_ms)-(caf*a*m*Speed_ms*Speed_ms*Speed_ms);
    Kg2 = (car*caf*L*L)+(m*Speed_ms*Speed_ms*(b*car-a*caf));
    KK_gain = Kg1/Kg2;
    Vy_SteerAngle_Kv = KK_gain*(SteerWheelAngle/15.5/57.3);
    %%  根据Vy/YawRate = KKK_gain
    KKK_gain = (b-(m*a*Speed_ms*Speed_ms)/(car*L));
    Vy_YawRate = (YawRate)*KKK_gain;
    %%  根据Vy/YawRate = KKK_gain,质心侧偏角为0时的，质心侧偏角的临界车速值，超过该车速质心侧偏角会反向，Vy也会反向
    Critical_Spd = sqrt((car*L*b)/(m*a));
    %%  由于前后轮胎刚度不确定，通常可时实际测得CharSpd，通过调整前后轮胎刚度使计算得到的车辆特征车速尽可能接近测试值，进而使设定的轮胎刚度更加接近真实值
    CharSpd= sqrt(1/((m/(L*L))*((b/caf)-(a/car)))); % 车辆特征车速（过渡转向和转向不足的临界车速，ESP提供）
    %% 转向性质表征 小于零为转向不足，大于零为转向过度
    SteerChar = sign(a*caf-b*car);
    %% 理论计算特征车速
    SM = abs(-((a*caf-b*car)/(L*(caf+car))));%静态裕度
    temp = (2*L*(caf/2)*(car/2))/(m*((caf/2)+(car/2)));
    Vch_Cal = sqrt(temp*(1/SM));
end
